simulink model "FeedBack_Linearization"  (R2021b)
settings: Solver=VariableStepAuto  StartTime=0.0  StopTime=10.0  RelTol=1e-3
undefined symbols (not defined in the file or in its folder): Kd, Kp, q_dq_init
(part 3 of 3)

== matlab function FeedBack_Linearization/G ==
  data: q input; G output; g input
function G = G(q,g)
%G_fun
%    G = G_fun(Q1,Q2,Q3,Q4,Q5,Q6,g)

%    This function was generated by the Symbolic Math Toolbox version 9.0.
%    28-Mar-2022 14:37:59

q1 = q(1);
q2 = q(2);
q3 = q(3);
q4 = q(4);
q5 = q(5);
q6 = q(6);

t2 = cos(q1);
t3 = cos(q2);
t4 = cos(q4);
t5 = cos(q5);
t6 = cos(q6);
t7 = sin(q1);
t8 = sin(q2);
t9 = sin(q4);
t10 = sin(q5);
t11 = sin(q6);
mt1 = [g.*t2.*(1.07e+2./1.0e+3)-g.*t7.*(3.0./5.0e+1)+g.*t3.*t7.*5.13502e-1+g.*t7.*t8.*1.895e-1+g.*q3.*t3.*t7.*(1.9e+1./5.0e+1)+g.*t3.*t5.*t7.*1.91e-4+(g.*t2.*t4.*t11)./1.0e+4-g.*t2.*t9.*t10.*1.91e-4+(g.*t3.*t5.*t6.*t7)./1.0e+4-(g.*t2.*t6.*t9.*t10)./1.0e+4-g.*t4.*t7.*t8.*t10.*1.91e-4-(g.*t7.*t8.*t9.*t11)./1.0e+4-(g.*t4.*t6.*t7.*t8.*t10)./1.0e+4];
mt2 = [g.*t2.*t3.*(-1.895e-1)+g.*t2.*t8.*5.13502e-1+g.*q3.*t2.*t8.*(1.9e+1./5.0e+1)+g.*t2.*t5.*t8.*1.91e-4+g.*t2.*t3.*t4.*t10.*1.91e-4+(g.*t2.*t5.*t6.*t8)./1.0e+4+(g.*t2.*t3.*t9.*t11)./1.0e+4+(g.*t2.*t3.*t4.*t6.*t10)./1.0e+4;g.*t2.*t3.*(-1.9e+1./5.0e+1)];
mt3 = [g.*t4.*t7.*t10.*(-1.91e-4)-(g.*t7.*t9.*t11)./1.0e+4+(g.*t2.*t4.*t8.*t11)./1.0e+4-(g.*t4.*t6.*t7.*t10)./1.0e+4-g.*t2.*t8.*t9.*t10.*1.91e-4-(g.*t2.*t6.*t8.*t9.*t10)./1.0e+4;g.*t2.*t3.*t10.*1.91e-4-g.*t5.*t7.*t9.*1.91e-4+g.*t2.*t4.*t5.*t8.*1.91e-4+(g.*t2.*t3.*t6.*t10)./1.0e+4-(g.*t5.*t6.*t7.*t9)./1.0e+4+(g.*t2.*t4.*t5.*t6.*t8)./1.0e+4];
mt4 = [(g.*t4.*t6.*t7)./1.0e+4+(g.*t2.*t3.*t5.*t11)./1.0e+4+(g.*t2.*t6.*t8.*t9)./1.0e+4+(g.*t7.*t9.*t10.*t11)./1.0e+4-(g.*t2.*t4.*t8.*t10.*t11)./1.0e+4];
G = [mt1;mt2;mt3;mt4];

== matlab function FeedBack_Linearization/Subsystem/Robot1 ==
  data: q_dq input; dq_ddq output; u input; q output; dq output; g input
function [dq_ddq,q,dq] = fcn(q_dq,u,g)
    q = q_dq(1:length(q_dq)/2);
    dq = q_dq(length(q_dq)/2+1:length(q_dq));
    g_num = g;

%     in1 = q;
%     in2 = [q;dq];
%     in3 = [q;g_num];
%     in1 = mat2cell(in1,ones(numel(in1),1),1);
%     in2 = mat2cell(in2,ones(numel(in2),1),1);
%     in3 = mat2cell(in3,ones(numel(in3),1),1);


    M = M_fun(q);
    C = C_fun(q,dq);
    G = G_fun(q,g_num);

    ddq = M\(u - C - G);
    
    dq_ddq = [dq;ddq];

end
